simulink model "ukl_ciagly_18"  (R2018b)
settings: Solver=VariableStepAuto  StartTime=0.0  StopTime=20  RelTol=1e-3
InitFcn:
  | T=0.001;
settings Model: Creator=Dominik  LastModifiedBy=user
settings SFSimCC: SimUseLocalCustomCode=off
settings RTWCC: RTWUseLocalCustomCode=off

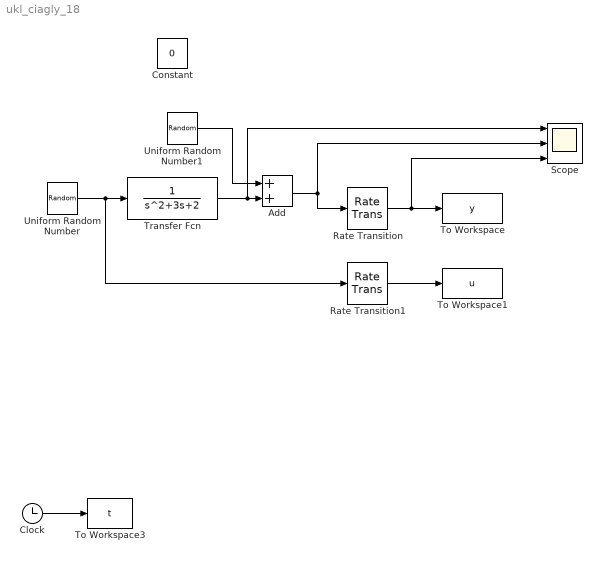
== system ukl_ciagly_18 ==
  Add : Sum
  Clock : Clock
  Constant : Constant  Value=0
  Rate Transition : RateTransition  OutPortSampleTime=T
  Rate Transition1 : RateTransition  OutPortSampleTime=T
  Scope : Scope  NumInputPorts=3
  To Workspace : ToWorkspace  VariableName=y  SampleTime=-1
  To Workspace1 : ToWorkspace  VariableName=u  SampleTime=-1
  To Workspace3 : ToWorkspace  VariableName=t  SampleTime=-1
  Transfer Fcn : TransferFcn  Denominator=[1 3 2]
  Uniform Random Number : UniformRandomNumber  SampleTime=T
  Uniform Random Number1 : UniformRandomNumber  Minimum=-0.00001  Maximum=0.00001  Seed=2422  SampleTime=T
  wires:
  Transfer Fcn/1 -> Scope/1, Add/2
  Uniform Random Number/1 -> Rate Transition1/1, Transfer Fcn/1
  Clock/1 -> To Workspace3/1
  Uniform Random Number1/1 -> Add/1
  Add/1 -> Scope/2, Rate Transition/1
  Rate Transition/1 -> Scope/3, To Workspace/1
  Rate Transition1/1 -> To Workspace1/1
